simulink model "FKtest2"  (Simulink 6.6)
settings: Solver=ode4  StartTime=0.0  StopTime=400  FixedStep=0.05  RelTol=1e-3
values from neighbouring files (symbols this model uses):
  vessel =     [input.mat]    (also in supply.mat)
libraries: marine_gnc x10, simulink x1
(part 2 of 2)

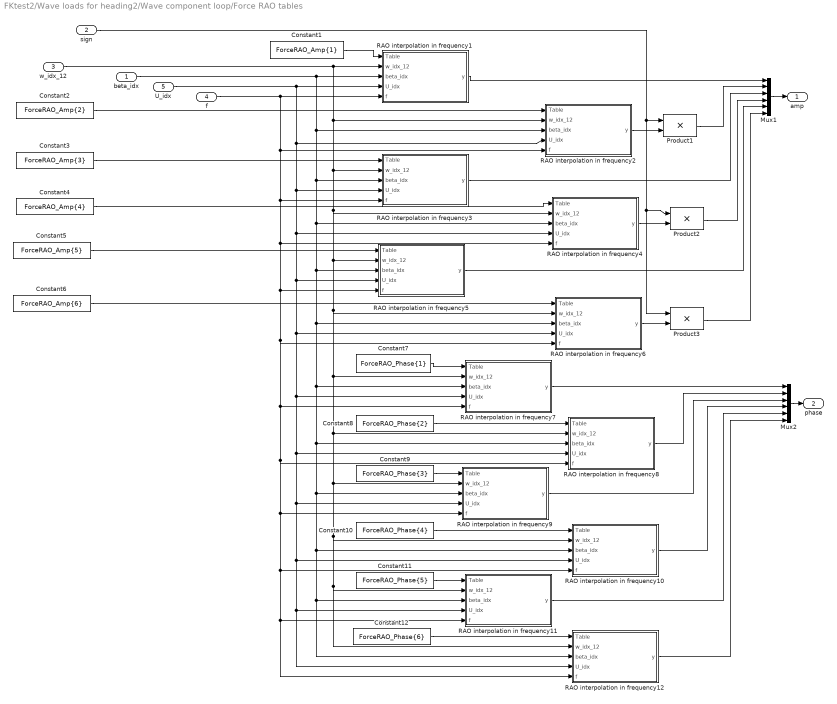
== system FKtest2/Wave loads for heading2/Wave component loop/Force RAO tables ==
  beta_idx : Inport
  sign : Inport  Port=2
  w_idx_12 : Inport  Port=3
  f : Inport  Port=4
  U_idx : Inport  Port=5
  Constant1 : Constant  Value=ForceRAO_Amp{1}
  Constant10 : Constant  Value=ForceRAO_Phase{4}
  Constant11 : Constant  Value=ForceRAO_Phase{5}
  Constant12 : Constant  Value=ForceRAO_Phase{6}
  Constant2 : Constant  Value=ForceRAO_Amp{2}
  Constant3 : Constant  Value=ForceRAO_Amp{3}
  Constant4 : Constant  Value=ForceRAO_Amp{4}
  Constant5 : Constant  Value=ForceRAO_Amp{5}
  Constant6 : Constant  Value=ForceRAO_Amp{6}
  Constant7 : Constant  Value=ForceRAO_Phase{1}
  Constant8 : Constant  Value=ForceRAO_Phase{2}
  Constant9 : Constant  Value=ForceRAO_Phase{3}
  Mux1 : Mux  Inputs=6
  Mux2 : Mux  Inputs=6
  Product1 : Product  Inputs=**  SaturateOnIntegerOverflow=on
  Product2 : Product  Inputs=**  SaturateOnIntegerOverflow=on
  Product3 : Product  Inputs=**  SaturateOnIntegerOverflow=on
  RAO interpolation in frequency1 : Subsystem
  RAO interpolation in frequency10 : Subsystem
  RAO interpolation in frequency11 : Subsystem
  RAO interpolation in frequency12 : Subsystem
  RAO interpolation in frequency2 : Subsystem
  RAO interpolation in frequency3 : Subsystem
  RAO interpolation in frequency4 : Subsystem
  RAO interpolation in frequency5 : Subsystem
  RAO interpolation in frequency6 : Subsystem
  RAO interpolation in frequency7 : Subsystem
  RAO interpolation in frequency8 : Subsystem
  RAO interpolation in frequency9 : Subsystem
  amp : Outport
  phase : Outport  Port=2
  wires:
  Mux1/1 -> amp/1
  Mux2/1 -> phase/1
  sign/1 -> Product3/1, Product2/1, Product1/1
  RAO interpolation in frequency6/1(y) -> Product3/2
  Product3/1 -> Mux1/6
  Product2/1 -> Mux1/4
  RAO interpolation in frequency2/1(y) -> Product1/2
  Product1/1 -> Mux1/2
  RAO interpolation in frequency5/1(y) -> Mux1/5
  RAO interpolation in frequency3/1(y) -> Mux1/3
  RAO interpolation in frequency1/1(y) -> Mux1/1
  Constant1/1 -> RAO interpolation in frequency1/1(Table)
  Constant2/1 -> RAO interpolation in frequency2/1(Table)
  Constant3/1 -> RAO interpolation in frequency3/1(Table)
  U_idx/1 -> RAO interpolation in frequency1/4(U_idx), RAO interpolation in frequency11/4(U_idx), RAO interpolation in frequency12/4(U_idx), RAO interpolation in frequency10/4(U_idx), RAO interpolation in frequency9/4(U_idx), RAO interpolation in frequency8/4(U_idx), RAO interpolation in frequency7/4(U_idx), RAO interpolation in frequency6/4(U_idx), RAO interpolation in frequency5/4(U_idx), RAO interpolation in frequency4/4(U_idx), RAO interpolation in frequency3/4(U_idx), RAO interpolation in frequency2/4(U_idx)
  Constant4/1 -> RAO interpolation in frequency4/1(Table)
  RAO interpolation in frequency4/1(y) -> Product2/2
  Constant5/1 -> RAO interpolation in frequency5/1(Table)
  Constant6/1 -> RAO interpolation in frequency6/1(Table)
  RAO interpolation in frequency12/1(y) -> Mux2/6
  RAO interpolation in frequency8/1(y) -> Mux2/2
  Constant8/1 -> RAO interpolation in frequency8/1(Table)
  Constant9/1 -> RAO interpolation in frequency9/1(Table)
  Constant10/1 -> RAO interpolation in frequency10/1(Table)
  RAO interpolation in frequency10/1(y) -> Mux2/4
  Constant11/1 -> RAO interpolation in frequency11/1(Table)
  Constant12/1 -> RAO interpolation in frequency12/1(Table)
  beta_idx/1 -> RAO interpolation in frequency11/3(beta_idx), RAO interpolation in frequency12/3(beta_idx), RAO interpolation in frequency10/3(beta_idx), RAO interpolation in frequency9/3(beta_idx), RAO interpolation in frequency8/3(beta_idx), RAO interpolation in frequency7/3(beta_idx), RAO interpolation in frequency6/3(beta_idx), RAO interpolation in frequency5/3(beta_idx), RAO interpolation in frequency4/3(beta_idx), RAO interpolation in frequency3/3(beta_idx), RAO interpolation in frequency2/3(beta_idx), RAO interpolation in frequency1/3(beta_idx)
  RAO interpolation in frequency7/1(y) -> Mux2/1
  RAO interpolation in frequency9/1(y) -> Mux2/3
  RAO interpolation in frequency11/1(y) -> Mux2/5
  w_idx_12/1 -> RAO interpolation in frequency1/2(w_idx_12), RAO interpolation in frequency2/2(w_idx_12), RAO interpolation in frequency3/2(w_idx_12), RAO interpolation in frequency4/2(w_idx_12), RAO interpolation in frequency5/2(w_idx_12), RAO interpolation in frequency6/2(w_idx_12), RAO interpolation in frequency7/2(w_idx_12), RAO interpolation in frequency8/2(w_idx_12), RAO interpolation in frequency9/2(w_idx_12), RAO interpolation in frequency10/2(w_idx_12), RAO interpolation in frequency11/2(w_idx_12), RAO interpolation in frequency12/2(w_idx_12)
  f/1 -> RAO interpolation in frequency1/5(f), RAO interpolation in frequency2/5(f), RAO interpolation in frequency3/5(f), RAO interpolation in frequency4/5(f), RAO interpolation in frequency5/5(f), RAO interpolation in frequency6/5(f), RAO interpolation in frequency7/5(f), RAO interpolation in frequency8/5(f), RAO interpolation in frequency9/5(f), RAO interpolation in frequency10/5(f), RAO interpolation in frequency11/5(f), RAO interpolation in frequency12/5(f)
  Constant7/1 -> RAO interpolation in frequency7/1(Table)

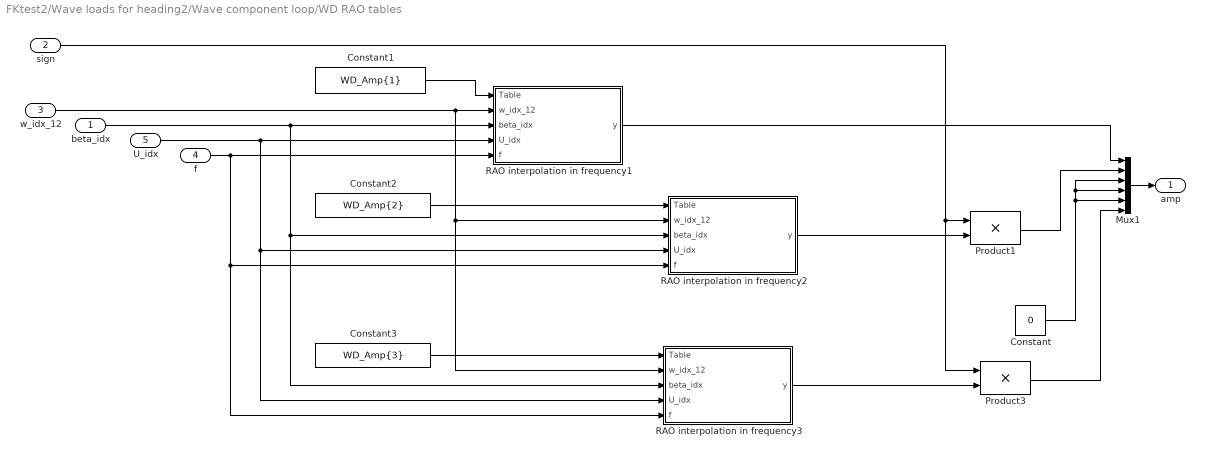
== system FKtest2/Wave loads for heading2/Wave component loop/WD RAO tables ==
  beta_idx : Inport
  sign : Inport  Port=2
  w_idx_12 : Inport  Port=3
  f : Inport  Port=4
  U_idx : Inport  Port=5
  Constant : Constant  Value=0
  Constant1 : Constant  Value=WD_Amp{1}
  Constant2 : Constant  Value=WD_Amp{2}
  Constant3 : Constant  Value=WD_Amp{3}
  Mux1 : Mux  Inputs=6
  Product1 : Product  Inputs=**  SaturateOnIntegerOverflow=on
  Product3 : Product  Inputs=**  SaturateOnIntegerOverflow=on
  RAO interpolation in frequency1 : Subsystem
  RAO interpolation in frequency2 : Subsystem
  RAO interpolation in frequency3 : Subsystem
  amp : Outport
  wires:
  Mux1/1 -> amp/1
  sign/1 -> Product1/1, Product3/1
  RAO interpolation in frequency3/1(y) -> Product3/2
  Product3/1 -> Mux1/6
  RAO interpolation in frequency2/1(y) -> Product1/2
  Product1/1 -> Mux1/2
  RAO interpolation in frequency1/1(y) -> Mux1/1
  Constant1/1 -> RAO interpolation in frequency1/1(Table)
  Constant2/1 -> RAO interpolation in frequency2/1(Table)
  U_idx/1 -> RAO interpolation in frequency2/4(U_idx), RAO interpolation in frequency3/4(U_idx), RAO interpolation in frequency1/4(U_idx)
  Constant3/1 -> RAO interpolation in frequency3/1(Table)
  beta_idx/1 -> RAO interpolation in frequency2/3(beta_idx), RAO interpolation in frequency3/3(beta_idx), RAO interpolation in frequency1/3(beta_idx)
  Constant/1 -> Mux1/3, Mux1/4, Mux1/5
  w_idx_12/1 -> RAO interpolation in frequency1/2(w_idx_12), RAO interpolation in frequency2/2(w_idx_12), RAO interpolation in frequency3/2(w_idx_12)
  f/1 -> RAO interpolation in frequency1/5(f), RAO interpolation in frequency2/5(f), RAO interpolation in frequency3/5(f)

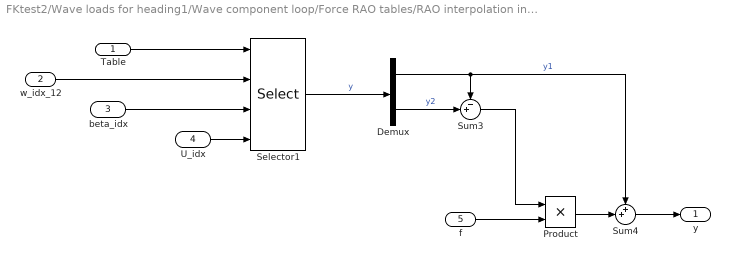
== system FKtest2/Wave loads for heading1/Wave component loop/Force RAO tables/RAO interpolation in frequency1 ==
  Table : Inport
  w_idx_12 : Inport  Port=2
  beta_idx : Inport  Port=3
  U_idx : Inport  Port=4
  f : Inport  Port=5
  Demux : Demux  Outputs=2
  Product : Product  RndMeth=Zero
  Selector1 : Selector  NumberOfDimensions=3  IndexOptions=Index vector (port),Index vector (port),Index vector (port)  Indices=[1 3],1,1  OutputSizes=1,1,1
  Sum3 : Sum  Inputs=-+|
  Sum4 : Sum  Inputs=++|
  y : Outport
  wires:
  Table/1 -> Selector1/1
  beta_idx/1 -> Selector1/3
  U_idx/1 -> Selector1/4
  Sum4/1 -> y/1
  Sum3/1 -> Product/1
  Product/1 -> Sum4/2
  Demux/1 -> Sum4/1, Sum3/1  "y1"
  Demux/2 -> Sum3/2  "y2"
  Selector1/1 -> Demux/1  "y"
  w_idx_12/1 -> Selector1/2
  f/1 -> Product/2

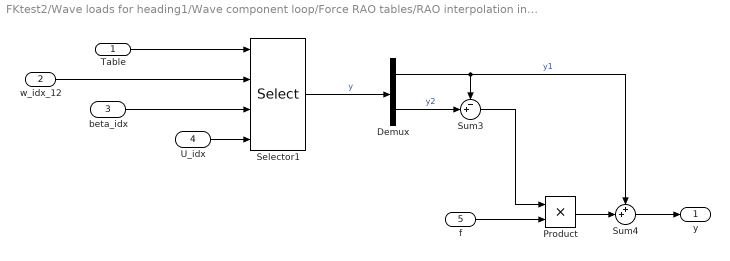
== system FKtest2/Wave loads for heading1/Wave component loop/Force RAO tables/RAO interpolation in frequency10 ==
  Table : Inport
  w_idx_12 : Inport  Port=2
  beta_idx : Inport  Port=3
  U_idx : Inport  Port=4
  f : Inport  Port=5
  Demux : Demux  Outputs=2
  Product : Product  RndMeth=Zero
  Selector1 : Selector  NumberOfDimensions=3  IndexOptions=Index vector (port),Index vector (port),Index vector (port)  Indices=[1 3],1,1  OutputSizes=1,1,1
  Sum3 : Sum  Inputs=-+|
  Sum4 : Sum  Inputs=++|
  y : Outport
  wires:
  Table/1 -> Selector1/1
  beta_idx/1 -> Selector1/3
  U_idx/1 -> Selector1/4
  Sum4/1 -> y/1
  Sum3/1 -> Product/1
  Product/1 -> Sum4/2
  Demux/1 -> Sum4/1, Sum3/1  "y1"
  Demux/2 -> Sum3/2  "y2"
  Selector1/1 -> Demux/1  "y"
  w_idx_12/1 -> Selector1/2
  f/1 -> Product/2

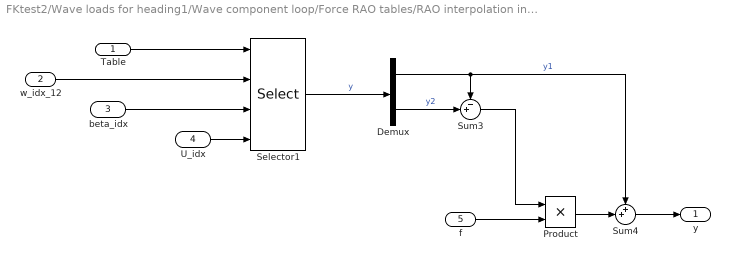
== system FKtest2/Wave loads for heading1/Wave component loop/Force RAO tables/RAO interpolation in frequency11 ==
  Table : Inport
  w_idx_12 : Inport  Port=2
  beta_idx : Inport  Port=3
  U_idx : Inport  Port=4
  f : Inport  Port=5
  Demux : Demux  Outputs=2
  Product : Product  RndMeth=Zero
  Selector1 : Selector  NumberOfDimensions=3  IndexOptions=Index vector (port),Index vector (port),Index vector (port)  Indices=[1 3],1,1  OutputSizes=1,1,1
  Sum3 : Sum  Inputs=-+|
  Sum4 : Sum  Inputs=++|
  y : Outport
  wires:
  Table/1 -> Selector1/1
  beta_idx/1 -> Selector1/3
  U_idx/1 -> Selector1/4
  Sum4/1 -> y/1
  Sum3/1 -> Product/1
  Product/1 -> Sum4/2
  Demux/1 -> Sum4/1, Sum3/1  "y1"
  Demux/2 -> Sum3/2  "y2"
  Selector1/1 -> Demux/1  "y"
  w_idx_12/1 -> Selector1/2
  f/1 -> Product/2

== system FKtest2/Wave loads for heading1/Wave component loop/Force RAO tables/RAO interpolation in frequency12 ==
  Table : Inport
  w_idx_12 : Inport  Port=2
  beta_idx : Inport  Port=3
  U_idx : Inport  Port=4
  f : Inport  Port=5
  Demux : Demux  Outputs=2
  Product : Product  RndMeth=Zero
  Selector1 : Selector  NumberOfDimensions=3  IndexOptions=Index vector (port),Index vector (port),Index vector (port)  Indices=[1 3],1,1  OutputSizes=1,1,1
  Sum3 : Sum  Inputs=-+|
  Sum4 : Sum  Inputs=++|
  y : Outport
  wires:
  Table/1 -> Selector1/1
  beta_idx/1 -> Selector1/3
  U_idx/1 -> Selector1/4
  Sum4/1 -> y/1
  Sum3/1 -> Product/1
  Product/1 -> Sum4/2
  Demux/1 -> Sum4/1, Sum3/1  "y1"
  Demux/2 -> Sum3/2  "y2"
  Selector1/1 -> Demux/1  "y"
  w_idx_12/1 -> Selector1/2
  f/1 -> Product/2

== system FKtest2/Wave loads for heading1/Wave component loop/Force RAO tables/RAO interpolation in frequency2 ==
  Table : Inport
  w_idx_12 : Inport  Port=2
  beta_idx : Inport  Port=3
  U_idx : Inport  Port=4
  f : Inport  Port=5
  Demux : Demux  Outputs=2
  Product : Product  RndMeth=Zero
  Selector1 : Selector  NumberOfDimensions=3  IndexOptions=Index vector (port),Index vector (port),Index vector (port)  Indices=[1 3],1,1  OutputSizes=1,1,1
  Sum3 : Sum  Inputs=-+|
  Sum4 : Sum  Inputs=++|
  y : Outport
  wires:
  Table/1 -> Selector1/1
  beta_idx/1 -> Selector1/3
  U_idx/1 -> Selector1/4
  Sum4/1 -> y/1
  Sum3/1 -> Product/1
  Product/1 -> Sum4/2
  Demux/1 -> Sum4/1, Sum3/1  "y1"
  Demux/2 -> Sum3/2  "y2"
  Selector1/1 -> Demux/1  "y"
  w_idx_12/1 -> Selector1/2
  f/1 -> Product/2

== system FKtest2/Wave loads for heading1/Wave component loop/Force RAO tables/RAO interpolation in frequency3 ==
  Table : Inport
  w_idx_12 : Inport  Port=2
  beta_idx : Inport  Port=3
  U_idx : Inport  Port=4
  f : Inport  Port=5
  Demux : Demux  Outputs=2
  Product : Product  RndMeth=Zero
  Selector1 : Selector  NumberOfDimensions=3  IndexOptions=Index vector (port),Index vector (port),Index vector (port)  Indices=[1 3],1,1  OutputSizes=1,1,1
  Sum3 : Sum  Inputs=-+|
  Sum4 : Sum  Inputs=++|
  y : Outport
  wires:
  Table/1 -> Selector1/1
  beta_idx/1 -> Selector1/3
  U_idx/1 -> Selector1/4
  Sum4/1 -> y/1
  Sum3/1 -> Product/1
  Product/1 -> Sum4/2
  Demux/1 -> Sum4/1, Sum3/1  "y1"
  Demux/2 -> Sum3/2  "y2"
  Selector1/1 -> Demux/1  "y"
  w_idx_12/1 -> Selector1/2
  f/1 -> Product/2

== system FKtest2/Wave loads for heading1/Wave component loop/Force RAO tables/RAO interpolation in frequency4 ==
  Table : Inport
  w_idx_12 : Inport  Port=2
  beta_idx : Inport  Port=3
  U_idx : Inport  Port=4
  f : Inport  Port=5
  Demux : Demux  Outputs=2
  Product : Product  RndMeth=Zero
  Selector1 : Selector  NumberOfDimensions=3  IndexOptions=Index vector (port),Index vector (port),Index vector (port)  Indices=[1 3],1,1  OutputSizes=1,1,1
  Sum3 : Sum  Inputs=-+|
  Sum4 : Sum  Inputs=++|
  y : Outport
  wires:
  Table/1 -> Selector1/1
  beta_idx/1 -> Selector1/3
  U_idx/1 -> Selector1/4
  Sum4/1 -> y/1
  Sum3/1 -> Product/1
  Product/1 -> Sum4/2
  Demux/1 -> Sum4/1, Sum3/1  "y1"
  Demux/2 -> Sum3/2  "y2"
  Selector1/1 -> Demux/1  "y"
  w_idx_12/1 -> Selector1/2
  f/1 -> Product/2

== system FKtest2/Wave loads for heading1/Wave component loop/Force RAO tables/RAO interpolation in frequency5 ==
  Table : Inport
  w_idx_12 : Inport  Port=2
  beta_idx : Inport  Port=3
  U_idx : Inport  Port=4
  f : Inport  Port=5
  Demux : Demux  Outputs=2
  Product : Product  RndMeth=Zero
  Selector1 : Selector  NumberOfDimensions=3  IndexOptions=Index vector (port),Index vector (port),Index vector (port)  Indices=[1 3],1,1  OutputSizes=1,1,1
  Sum3 : Sum  Inputs=-+|
  Sum4 : Sum  Inputs=++|
  y : Outport
  wires:
  Table/1 -> Selector1/1
  beta_idx/1 -> Selector1/3
  U_idx/1 -> Selector1/4
  Sum4/1 -> y/1
  Sum3/1 -> Product/1
  Product/1 -> Sum4/2
  Demux/1 -> Sum4/1, Sum3/1  "y1"
  Demux/2 -> Sum3/2  "y2"
  Selector1/1 -> Demux/1  "y"
  w_idx_12/1 -> Selector1/2
  f/1 -> Product/2

== system FKtest2/Wave loads for heading1/Wave component loop/Force RAO tables/RAO interpolation in frequency6 ==
  Table : Inport
  w_idx_12 : Inport  Port=2
  beta_idx : Inport  Port=3
  U_idx : Inport  Port=4
  f : Inport  Port=5
  Demux : Demux  Outputs=2
  Product : Product  RndMeth=Zero
  Selector1 : Selector  NumberOfDimensions=3  IndexOptions=Index vector (port),Index vector (port),Index vector (port)  Indices=[1 3],1,1  OutputSizes=1,1,1
  Sum3 : Sum  Inputs=-+|
  Sum4 : Sum  Inputs=++|
  y : Outport
  wires:
  Table/1 -> Selector1/1
  beta_idx/1 -> Selector1/3
  U_idx/1 -> Selector1/4
  Sum4/1 -> y/1
  Sum3/1 -> Product/1
  Product/1 -> Sum4/2
  Demux/1 -> Sum4/1, Sum3/1  "y1"
  Demux/2 -> Sum3/2  "y2"
  Selector1/1 -> Demux/1  "y"
  w_idx_12/1 -> Selector1/2
  f/1 -> Product/2

== system FKtest2/Wave loads for heading1/Wave component loop/Force RAO tables/RAO interpolation in frequency7 ==
  Table : Inport
  w_idx_12 : Inport  Port=2
  beta_idx : Inport  Port=3
  U_idx : Inport  Port=4
  f : Inport  Port=5
  Demux : Demux  Outputs=2
  Product : Product  RndMeth=Zero
  Selector1 : Selector  NumberOfDimensions=3  IndexOptions=Index vector (port),Index vector (port),Index vector (port)  Indices=[1 3],1,1  OutputSizes=1,1,1
  Sum3 : Sum  Inputs=-+|
  Sum4 : Sum  Inputs=++|
  y : Outport
  wires:
  Table/1 -> Selector1/1
  beta_idx/1 -> Selector1/3
  U_idx/1 -> Selector1/4
  Sum4/1 -> y/1
  Sum3/1 -> Product/1
  Product/1 -> Sum4/2
  Demux/1 -> Sum4/1, Sum3/1  "y1"
  Demux/2 -> Sum3/2  "y2"
  Selector1/1 -> Demux/1  "y"
  w_idx_12/1 -> Selector1/2
  f/1 -> Product/2

== system FKtest2/Wave loads for heading1/Wave component loop/Force RAO tables/RAO interpolation in frequency8 ==
  Table : Inport
  w_idx_12 : Inport  Port=2
  beta_idx : Inport  Port=3
  U_idx : Inport  Port=4
  f : Inport  Port=5
  Demux : Demux  Outputs=2
  Product : Product  RndMeth=Zero
  Selector1 : Selector  NumberOfDimensions=3  IndexOptions=Index vector (port),Index vector (port),Index vector (port)  Indices=[1 3],1,1  OutputSizes=1,1,1
  Sum3 : Sum  Inputs=-+|
  Sum4 : Sum  Inputs=++|
  y : Outport
  wires:
  Table/1 -> Selector1/1
  beta_idx/1 -> Selector1/3
  U_idx/1 -> Selector1/4
  Sum4/1 -> y/1
  Sum3/1 -> Product/1
  Product/1 -> Sum4/2
  Demux/1 -> Sum4/1, Sum3/1  "y1"
  Demux/2 -> Sum3/2  "y2"
  Selector1/1 -> Demux/1  "y"
  w_idx_12/1 -> Selector1/2
  f/1 -> Product/2

== system FKtest2/Wave loads for heading1/Wave component loop/Force RAO tables/RAO interpolation in frequency9 ==
  Table : Inport
  w_idx_12 : Inport  Port=2
  beta_idx : Inport  Port=3
  U_idx : Inport  Port=4
  f : Inport  Port=5
  Demux : Demux  Outputs=2
  Product : Product  RndMeth=Zero
  Selector1 : Selector  NumberOfDimensions=3  IndexOptions=Index vector (port),Index vector (port),Index vector (port)  Indices=[1 3],1,1  OutputSizes=1,1,1
  Sum3 : Sum  Inputs=-+|
  Sum4 : Sum  Inputs=++|
  y : Outport
  wires:
  Table/1 -> Selector1/1
  beta_idx/1 -> Selector1/3
  U_idx/1 -> Selector1/4
  Sum4/1 -> y/1
  Sum3/1 -> Product/1
  Product/1 -> Sum4/2
  Demux/1 -> Sum4/1, Sum3/1  "y1"
  Demux/2 -> Sum3/2  "y2"
  Selector1/1 -> Demux/1  "y"
  w_idx_12/1 -> Selector1/2
  f/1 -> Product/2

== system FKtest2/Wave loads for heading1/Wave component loop/WD RAO tables/RAO interpolation in frequency1 ==
  Table : Inport
  w_idx_12 : Inport  Port=2
  beta_idx : Inport  Port=3
  U_idx : Inport  Port=4
  f : Inport  Port=5
  Demux : Demux  Outputs=2
  Product : Product  RndMeth=Zero
  Selector1 : Selector  NumberOfDimensions=3  IndexOptions=Index vector (port),Index vector (port),Index vector (port)  Indices=[1 3],1,1  OutputSizes=1,1,1
  Sum3 : Sum  Inputs=-+|
  Sum4 : Sum  Inputs=++|
  y : Outport
  wires:
  Table/1 -> Selector1/1
  beta_idx/1 -> Selector1/3
  U_idx/1 -> Selector1/4
  Sum4/1 -> y/1
  Sum3/1 -> Product/1
  Product/1 -> Sum4/2
  Demux/1 -> Sum4/1, Sum3/1  "y1"
  Demux/2 -> Sum3/2  "y2"
  Selector1/1 -> Demux/1  "y"
  w_idx_12/1 -> Selector1/2
  f/1 -> Product/2

== system FKtest2/Wave loads for heading1/Wave component loop/WD RAO tables/RAO interpolation in frequency2 ==
  Table : Inport
  w_idx_12 : Inport  Port=2
  beta_idx : Inport  Port=3
  U_idx : Inport  Port=4
  f : Inport  Port=5
  Demux : Demux  Outputs=2
  Product : Product  RndMeth=Zero
  Selector1 : Selector  NumberOfDimensions=3  IndexOptions=Index vector (port),Index vector (port),Index vector (port)  Indices=[1 3],1,1  OutputSizes=1,1,1
  Sum3 : Sum  Inputs=-+|
  Sum4 : Sum  Inputs=++|
  y : Outport
  wires:
  Table/1 -> Selector1/1
  beta_idx/1 -> Selector1/3
  U_idx/1 -> Selector1/4
  Sum4/1 -> y/1
  Sum3/1 -> Product/1
  Product/1 -> Sum4/2
  Demux/1 -> Sum4/1, Sum3/1  "y1"
  Demux/2 -> Sum3/2  "y2"
  Selector1/1 -> Demux/1  "y"
  w_idx_12/1 -> Selector1/2
  f/1 -> Product/2

== system FKtest2/Wave loads for heading1/Wave component loop/WD RAO tables/RAO interpolation in frequency3 ==
  Table : Inport
  w_idx_12 : Inport  Port=2
  beta_idx : Inport  Port=3
  U_idx : Inport  Port=4
  f : Inport  Port=5
  Demux : Demux  Outputs=2
  Product : Product  RndMeth=Zero
  Selector1 : Selector  NumberOfDimensions=3  IndexOptions=Index vector (port),Index vector (port),Index vector (port)  Indices=[1 3],1,1  OutputSizes=1,1,1
  Sum3 : Sum  Inputs=-+|
  Sum4 : Sum  Inputs=++|
  y : Outport
  wires:
  Table/1 -> Selector1/1
  beta_idx/1 -> Selector1/3
  U_idx/1 -> Selector1/4
  Sum4/1 -> y/1
  Sum3/1 -> Product/1
  Product/1 -> Sum4/2
  Demux/1 -> Sum4/1, Sum3/1  "y1"
  Demux/2 -> Sum3/2  "y2"
  Selector1/1 -> Demux/1  "y"
  w_idx_12/1 -> Selector1/2
  f/1 -> Product/2

== system FKtest2/Wave loads for heading2/Wave component loop/Force RAO tables/RAO interpolation in frequency1 ==
  Table : Inport
  w_idx_12 : Inport  Port=2
  beta_idx : Inport  Port=3
  U_idx : Inport  Port=4
  f : Inport  Port=5
  Demux : Demux  Outputs=2
  Product : Product  RndMeth=Zero
  Selector1 : Selector  NumberOfDimensions=3  IndexOptions=Index vector (port),Index vector (port),Index vector (port)  Indices=[1 3],1,1  OutputSizes=1,1,1
  Sum3 : Sum  Inputs=-+|
  Sum4 : Sum  Inputs=++|
  y : Outport
  wires:
  Table/1 -> Selector1/1
  beta_idx/1 -> Selector1/3
  U_idx/1 -> Selector1/4
  Sum4/1 -> y/1
  Sum3/1 -> Product/1
  Product/1 -> Sum4/2
  Demux/1 -> Sum4/1, Sum3/1  "y1"
  Demux/2 -> Sum3/2  "y2"
  Selector1/1 -> Demux/1  "y"
  w_idx_12/1 -> Selector1/2
  f/1 -> Product/2

== system FKtest2/Wave loads for heading2/Wave component loop/Force RAO tables/RAO interpolation in frequency10 ==
  Table : Inport
  w_idx_12 : Inport  Port=2
  beta_idx : Inport  Port=3
  U_idx : Inport  Port=4
  f : Inport  Port=5
  Demux : Demux  Outputs=2
  Product : Product  RndMeth=Zero
  Selector1 : Selector  NumberOfDimensions=3  IndexOptions=Index vector (port),Index vector (port),Index vector (port)  Indices=[1 3],1,1  OutputSizes=1,1,1
  Sum3 : Sum  Inputs=-+|
  Sum4 : Sum  Inputs=++|
  y : Outport
  wires:
  Table/1 -> Selector1/1
  beta_idx/1 -> Selector1/3
  U_idx/1 -> Selector1/4
  Sum4/1 -> y/1
  Sum3/1 -> Product/1
  Product/1 -> Sum4/2
  Demux/1 -> Sum4/1, Sum3/1  "y1"
  Demux/2 -> Sum3/2  "y2"
  Selector1/1 -> Demux/1  "y"
  w_idx_12/1 -> Selector1/2
  f/1 -> Product/2

== system FKtest2/Wave loads for heading2/Wave component loop/Force RAO tables/RAO interpolation in frequency11 ==
  Table : Inport
  w_idx_12 : Inport  Port=2
  beta_idx : Inport  Port=3
  U_idx : Inport  Port=4
  f : Inport  Port=5
  Demux : Demux  Outputs=2
  Product : Product  RndMeth=Zero
  Selector1 : Selector  NumberOfDimensions=3  IndexOptions=Index vector (port),Index vector (port),Index vector (port)  Indices=[1 3],1,1  OutputSizes=1,1,1
  Sum3 : Sum  Inputs=-+|
  Sum4 : Sum  Inputs=++|
  y : Outport
  wires:
  Table/1 -> Selector1/1
  beta_idx/1 -> Selector1/3
  U_idx/1 -> Selector1/4
  Sum4/1 -> y/1
  Sum3/1 -> Product/1
  Product/1 -> Sum4/2
  Demux/1 -> Sum4/1, Sum3/1  "y1"
  Demux/2 -> Sum3/2  "y2"
  Selector1/1 -> Demux/1  "y"
  w_idx_12/1 -> Selector1/2
  f/1 -> Product/2

== system FKtest2/Wave loads for heading2/Wave component loop/Force RAO tables/RAO interpolation in frequency12 ==
  Table : Inport
  w_idx_12 : Inport  Port=2
  beta_idx : Inport  Port=3
  U_idx : Inport  Port=4
  f : Inport  Port=5
  Demux : Demux  Outputs=2
  Product : Product  RndMeth=Zero
  Selector1 : Selector  NumberOfDimensions=3  IndexOptions=Index vector (port),Index vector (port),Index vector (port)  Indices=[1 3],1,1  OutputSizes=1,1,1
  Sum3 : Sum  Inputs=-+|
  Sum4 : Sum  Inputs=++|
  y : Outport
  wires:
  Table/1 -> Selector1/1
  beta_idx/1 -> Selector1/3
  U_idx/1 -> Selector1/4
  Sum4/1 -> y/1
  Sum3/1 -> Product/1
  Product/1 -> Sum4/2
  Demux/1 -> Sum4/1, Sum3/1  "y1"
  Demux/2 -> Sum3/2  "y2"
  Selector1/1 -> Demux/1  "y"
  w_idx_12/1 -> Selector1/2
  f/1 -> Product/2

== system FKtest2/Wave loads for heading2/Wave component loop/Force RAO tables/RAO interpolation in frequency2 ==
  Table : Inport
  w_idx_12 : Inport  Port=2
  beta_idx : Inport  Port=3
  U_idx : Inport  Port=4
  f : Inport  Port=5
  Demux : Demux  Outputs=2
  Product : Product  RndMeth=Zero
  Selector1 : Selector  NumberOfDimensions=3  IndexOptions=Index vector (port),Index vector (port),Index vector (port)  Indices=[1 3],1,1  OutputSizes=1,1,1
  Sum3 : Sum  Inputs=-+|
  Sum4 : Sum  Inputs=++|
  y : Outport
  wires:
  Table/1 -> Selector1/1
  beta_idx/1 -> Selector1/3
  U_idx/1 -> Selector1/4
  Sum4/1 -> y/1
  Sum3/1 -> Product/1
  Product/1 -> Sum4/2
  Demux/1 -> Sum4/1, Sum3/1  "y1"
  Demux/2 -> Sum3/2  "y2"
  Selector1/1 -> Demux/1  "y"
  w_idx_12/1 -> Selector1/2
  f/1 -> Product/2

== system FKtest2/Wave loads for heading2/Wave component loop/Force RAO tables/RAO interpolation in frequency3 ==
  Table : Inport
  w_idx_12 : Inport  Port=2
  beta_idx : Inport  Port=3
  U_idx : Inport  Port=4
  f : Inport  Port=5
  Demux : Demux  Outputs=2
  Product : Product  RndMeth=Zero
  Selector1 : Selector  NumberOfDimensions=3  IndexOptions=Index vector (port),Index vector (port),Index vector (port)  Indices=[1 3],1,1  OutputSizes=1,1,1
  Sum3 : Sum  Inputs=-+|
  Sum4 : Sum  Inputs=++|
  y : Outport
  wires:
  Table/1 -> Selector1/1
  beta_idx/1 -> Selector1/3
  U_idx/1 -> Selector1/4
  Sum4/1 -> y/1
  Sum3/1 -> Product/1
  Product/1 -> Sum4/2
  Demux/1 -> Sum4/1, Sum3/1  "y1"
  Demux/2 -> Sum3/2  "y2"
  Selector1/1 -> Demux/1  "y"
  w_idx_12/1 -> Selector1/2
  f/1 -> Product/2

== system FKtest2/Wave loads for heading2/Wave component loop/Force RAO tables/RAO interpolation in frequency4 ==
  Table : Inport
  w_idx_12 : Inport  Port=2
  beta_idx : Inport  Port=3
  U_idx : Inport  Port=4
  f : Inport  Port=5
  Demux : Demux  Outputs=2
  Product : Product  RndMeth=Zero
  Selector1 : Selector  NumberOfDimensions=3  IndexOptions=Index vector (port),Index vector (port),Index vector (port)  Indices=[1 3],1,1  OutputSizes=1,1,1
  Sum3 : Sum  Inputs=-+|
  Sum4 : Sum  Inputs=++|
  y : Outport
  wires:
  Table/1 -> Selector1/1
  beta_idx/1 -> Selector1/3
  U_idx/1 -> Selector1/4
  Sum4/1 -> y/1
  Sum3/1 -> Product/1
  Product/1 -> Sum4/2
  Demux/1 -> Sum4/1, Sum3/1  "y1"
  Demux/2 -> Sum3/2  "y2"
  Selector1/1 -> Demux/1  "y"
  w_idx_12/1 -> Selector1/2
  f/1 -> Product/2

== system FKtest2/Wave loads for heading2/Wave component loop/Force RAO tables/RAO interpolation in frequency5 ==
  Table : Inport
  w_idx_12 : Inport  Port=2
  beta_idx : Inport  Port=3
  U_idx : Inport  Port=4
  f : Inport  Port=5
  Demux : Demux  Outputs=2
  Product : Product  RndMeth=Zero
  Selector1 : Selector  NumberOfDimensions=3  IndexOptions=Index vector (port),Index vector (port),Index vector (port)  Indices=[1 3],1,1  OutputSizes=1,1,1
  Sum3 : Sum  Inputs=-+|
  Sum4 : Sum  Inputs=++|
  y : Outport
  wires:
  Table/1 -> Selector1/1
  beta_idx/1 -> Selector1/3
  U_idx/1 -> Selector1/4
  Sum4/1 -> y/1
  Sum3/1 -> Product/1
  Product/1 -> Sum4/2
  Demux/1 -> Sum4/1, Sum3/1  "y1"
  Demux/2 -> Sum3/2  "y2"
  Selector1/1 -> Demux/1  "y"
  w_idx_12/1 -> Selector1/2
  f/1 -> Product/2

== system FKtest2/Wave loads for heading2/Wave component loop/Force RAO tables/RAO interpolation in frequency6 ==
  Table : Inport
  w_idx_12 : Inport  Port=2
  beta_idx : Inport  Port=3
  U_idx : Inport  Port=4
  f : Inport  Port=5
  Demux : Demux  Outputs=2
  Product : Product  RndMeth=Zero
  Selector1 : Selector  NumberOfDimensions=3  IndexOptions=Index vector (port),Index vector (port),Index vector (port)  Indices=[1 3],1,1  OutputSizes=1,1,1
  Sum3 : Sum  Inputs=-+|
  Sum4 : Sum  Inputs=++|
  y : Outport
  wires:
  Table/1 -> Selector1/1
  beta_idx/1 -> Selector1/3
  U_idx/1 -> Selector1/4
  Sum4/1 -> y/1
  Sum3/1 -> Product/1
  Product/1 -> Sum4/2
  Demux/1 -> Sum4/1, Sum3/1  "y1"
  Demux/2 -> Sum3/2  "y2"
  Selector1/1 -> Demux/1  "y"
  w_idx_12/1 -> Selector1/2
  f/1 -> Product/2

== system FKtest2/Wave loads for heading2/Wave component loop/Force RAO tables/RAO interpolation in frequency7 ==
  Table : Inport
  w_idx_12 : Inport  Port=2
  beta_idx : Inport  Port=3
  U_idx : Inport  Port=4
  f : Inport  Port=5
  Demux : Demux  Outputs=2
  Product : Product  RndMeth=Zero
  Selector1 : Selector  NumberOfDimensions=3  IndexOptions=Index vector (port),Index vector (port),Index vector (port)  Indices=[1 3],1,1  OutputSizes=1,1,1
  Sum3 : Sum  Inputs=-+|
  Sum4 : Sum  Inputs=++|
  y : Outport
  wires:
  Table/1 -> Selector1/1
  beta_idx/1 -> Selector1/3
  U_idx/1 -> Selector1/4
  Sum4/1 -> y/1
  Sum3/1 -> Product/1
  Product/1 -> Sum4/2
  Demux/1 -> Sum4/1, Sum3/1  "y1"
  Demux/2 -> Sum3/2  "y2"
  Selector1/1 -> Demux/1  "y"
  w_idx_12/1 -> Selector1/2
  f/1 -> Product/2

== system FKtest2/Wave loads for heading2/Wave component loop/Force RAO tables/RAO interpolation in frequency8 ==
  Table : Inport
  w_idx_12 : Inport  Port=2
  beta_idx : Inport  Port=3
  U_idx : Inport  Port=4
  f : Inport  Port=5
  Demux : Demux  Outputs=2
  Product : Product  RndMeth=Zero
  Selector1 : Selector  NumberOfDimensions=3  IndexOptions=Index vector (port),Index vector (port),Index vector (port)  Indices=[1 3],1,1  OutputSizes=1,1,1
  Sum3 : Sum  Inputs=-+|
  Sum4 : Sum  Inputs=++|
  y : Outport
  wires:
  Table/1 -> Selector1/1
  beta_idx/1 -> Selector1/3
  U_idx/1 -> Selector1/4
  Sum4/1 -> y/1
  Sum3/1 -> Product/1
  Product/1 -> Sum4/2
  Demux/1 -> Sum4/1, Sum3/1  "y1"
  Demux/2 -> Sum3/2  "y2"
  Selector1/1 -> Demux/1  "y"
  w_idx_12/1 -> Selector1/2
  f/1 -> Product/2

== system FKtest2/Wave loads for heading2/Wave component loop/Force RAO tables/RAO interpolation in frequency9 ==
  Table : Inport
  w_idx_12 : Inport  Port=2
  beta_idx : Inport  Port=3
  U_idx : Inport  Port=4
  f : Inport  Port=5
  Demux : Demux  Outputs=2
  Product : Product  RndMeth=Zero
  Selector1 : Selector  NumberOfDimensions=3  IndexOptions=Index vector (port),Index vector (port),Index vector (port)  Indices=[1 3],1,1  OutputSizes=1,1,1
  Sum3 : Sum  Inputs=-+|
  Sum4 : Sum  Inputs=++|
  y : Outport
  wires:
  Table/1 -> Selector1/1
  beta_idx/1 -> Selector1/3
  U_idx/1 -> Selector1/4
  Sum4/1 -> y/1
  Sum3/1 -> Product/1
  Product/1 -> Sum4/2
  Demux/1 -> Sum4/1, Sum3/1  "y1"
  Demux/2 -> Sum3/2  "y2"
  Selector1/1 -> Demux/1  "y"
  w_idx_12/1 -> Selector1/2
  f/1 -> Product/2

== system FKtest2/Wave loads for heading2/Wave component loop/WD RAO tables/RAO interpolation in frequency1 ==
  Table : Inport
  w_idx_12 : Inport  Port=2
  beta_idx : Inport  Port=3
  U_idx : Inport  Port=4
  f : Inport  Port=5
  Demux : Demux  Outputs=2
  Product : Product  RndMeth=Zero
  Selector1 : Selector  NumberOfDimensions=3  IndexOptions=Index vector (port),Index vector (port),Index vector (port)  Indices=[1 3],1,1  OutputSizes=1,1,1
  Sum3 : Sum  Inputs=-+|
  Sum4 : Sum  Inputs=++|
  y : Outport
  wires:
  Table/1 -> Selector1/1
  beta_idx/1 -> Selector1/3
  U_idx/1 -> Selector1/4
  Sum4/1 -> y/1
  Sum3/1 -> Product/1
  Product/1 -> Sum4/2
  Demux/1 -> Sum4/1, Sum3/1  "y1"
  Demux/2 -> Sum3/2  "y2"
  Selector1/1 -> Demux/1  "y"
  w_idx_12/1 -> Selector1/2
  f/1 -> Product/2

== system FKtest2/Wave loads for heading2/Wave component loop/WD RAO tables/RAO interpolation in frequency2 ==
  Table : Inport
  w_idx_12 : Inport  Port=2
  beta_idx : Inport  Port=3
  U_idx : Inport  Port=4
  f : Inport  Port=5
  Demux : Demux  Outputs=2
  Product : Product  RndMeth=Zero
  Selector1 : Selector  NumberOfDimensions=3  IndexOptions=Index vector (port),Index vector (port),Index vector (port)  Indices=[1 3],1,1  OutputSizes=1,1,1
  Sum3 : Sum  Inputs=-+|
  Sum4 : Sum  Inputs=++|
  y : Outport
  wires:
  Table/1 -> Selector1/1
  beta_idx/1 -> Selector1/3
  U_idx/1 -> Selector1/4
  Sum4/1 -> y/1
  Sum3/1 -> Product/1
  Product/1 -> Sum4/2
  Demux/1 -> Sum4/1, Sum3/1  "y1"
  Demux/2 -> Sum3/2  "y2"
  Selector1/1 -> Demux/1  "y"
  w_idx_12/1 -> Selector1/2
  f/1 -> Product/2

== system FKtest2/Wave loads for heading2/Wave component loop/WD RAO tables/RAO interpolation in frequency3 ==
  Table : Inport
  w_idx_12 : Inport  Port=2
  beta_idx : Inport  Port=3
  U_idx : Inport  Port=4
  f : Inport  Port=5
  Demux : Demux  Outputs=2
  Product : Product  RndMeth=Zero
  Selector1 : Selector  NumberOfDimensions=3  IndexOptions=Index vector (port),Index vector (port),Index vector (port)  Indices=[1 3],1,1  OutputSizes=1,1,1
  Sum3 : Sum  Inputs=-+|
  Sum4 : Sum  Inputs=++|
  y : Outport
  wires:
  Table/1 -> Selector1/1
  beta_idx/1 -> Selector1/3
  U_idx/1 -> Selector1/4
  Sum4/1 -> y/1
  Sum3/1 -> Product/1
  Product/1 -> Sum4/2
  Demux/1 -> Sum4/1, Sum3/1  "y1"
  Demux/2 -> Sum3/2  "y2"
  Selector1/1 -> Demux/1  "y"
  w_idx_12/1 -> Selector1/2
  f/1 -> Product/2
